simulink model "LOS_depth"  (R2016b)
settings: Solver=VariableStepAuto  StartTime=0.0  StopTime=10.0  RelTol=1e-3
settings Model: Creator=Admin  LastModifiedBy=Admin

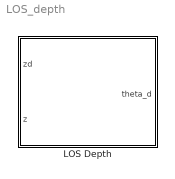
== system LOS_depth ==
  LOS Depth : MATLAB Function  TreatAsAtomicUnit=on

== matlab function LOS_depth/LOS Depth ==
  data: zd input; theta_d output; z input
function theta_d  = Calc_Ref(zd,z)
ze = z - zd;

delta_max = 5;
delta_min = 2.5;
K         = 0.7;
delta     = (delta_max - delta_min)*exp(-K*(ze)^2)+delta_min;
theta_d   = atan(ze/delta);
